simulink model "Buck_Boost_Converter"  (R2018a)
settings: Solver=VariableStepAuto  StartTime=0.0  StopTime=0.0003  RelTol=1e-3
libraries: powerlib x9
settings Model: Creator=SANDEEP GOWRAVAM  LastModifiedBy=SANDEEP GOWRAVAM

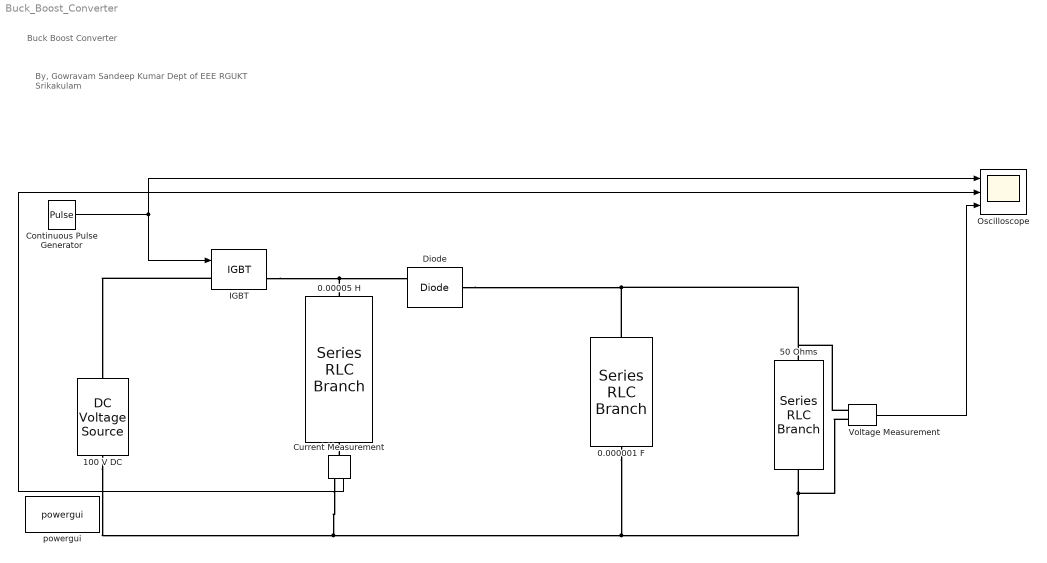
== system Buck_Boost_Converter ==
  note: By,
      | Gowravam Sandeep Kumar
      | Dept of EEE
      | RGUKT Srikakulam
  note: Buck Boost Converter
  "0.000001 F " : powerlib/Elements/Series RLC Branch  LConnTagsString=__new0  RConnTagsString=__new0  BranchType=C  Resistance=1  Inductance=1e-3  SetiL0=off  InitialCurrent=0  Capacitance=0.000001  Setx0=off  InitialVoltage=0  Measurements=None
  0.00005 H : powerlib/Elements/Series RLC Branch  LConnTagsString=__new0  RConnTagsString=__new0  BranchType=L  Resistance=1  Inductance=0.00005  SetiL0=off  InitialCurrent=0  Capacitance=1e-6  Setx0=off  InitialVoltage=0  Measurements=None
  100 V DC : powerlib/Electrical Sources/DC Voltage Source  Amplitude=100  Measurements=None
  50 Ohms : powerlib/Elements/Series RLC Branch  LConnTagsString=__new0  RConnTagsString=__new0  BranchType=R  Resistance=50  Inductance=1e-3  SetiL0=off  InitialCurrent=0  Capacitance=1e-6  Setx0=off  InitialVoltage=0  Measurements=None
  Continuous Pulse Generator : DiscretePulseGenerator  PulseType=Time based  Amplitude=2  Period=1/25000  PulseWidth=50
  Current Measurement : powerlib/Measurements/Current Measurement  PhasorSimulation=off  OutputType=Complex  PSBequivalent=0
  Diode : powerlib/Power Electronics/Diode  Ron=0.001  Lon=0  Vf=0.8  IC=0  UseSnubber=0  Rs=500  Cs=250e-9  Measurements=on
  IGBT : powerlib/Power Electronics/IGBT  Ron=0.001  Lon=0  Vf=1  Tf=1e-6  Tt=2e-6  IC=0  Rs=1e5  Cs=inf  Measurements=on
  Oscilloscope : Scope  NumInputPorts=3
  Voltage Measurement : powerlib/Measurements/Voltage Measurement  PhasorSimulation=off  OutputType=Complex  PSBequivalent=0
  powergui : powerlib/powergui  Priority=1  SimulationMode=Continuous  SampleTime=50e-6  frequency=60  Iterations=50  frequencyindice=0  Pbase=100e6  ErrMax=1e-4  UnitsV=kV  UnitsW=MW  buscounter=0  FunctionMessages=off  echomessages=off  EnableUseOfTLC=off  CurrentSourceSwitches=off  DisableSnubberDevices=off  DisableRonSwitches=off  DisableVfSwitches=off  DisplayEquations=off  SolverType=Tustin/Backward Euler (TBE)  Interpol=off  ExternalGateDelay=off  methode=off  Ts=100  x0status=blocks  SPID=on  SwTol=0  HookPort=off  RestoreLinks=warning  ResistiveCurrentMeasurement=off  Frange=[0:2:500]  Ylog=off  Xlog=on  ShowGrid=off  save=off  variable=ZData  structure=0  ZoomFFT=off  StartTime=0.0  cycles=1  DisplayStyle=1  fundamental=60  FreqAxis=off  MaxFrequency=1000  frequencyindicesteady=1  RmsSteady=1  display=off
  wires:
  Current Measurement/1 -> Oscilloscope/2
  Continuous Pulse Generator/1 -> IGBT/1, Oscilloscope/1
  Voltage Measurement/1 -> Oscilloscope/3
  connections:
  Diode/LConn1 -- "0.000001 F "/RConn1 -- Voltage Measurement/LConn1 -- 50 Ohms/LConn1
  100 V DC/LConn1 -- Current Measurement/RConn1 -- "0.000001 F "/LConn1 -- Voltage Measurement/LConn2 -- 50 Ohms/RConn1
  IGBT/LConn1 -- 100 V DC/RConn1
  0.00005 H/LConn1 -- Diode/RConn1 -- IGBT/RConn1
  Current Measurement/LConn1 -- 0.00005 H/RConn1
